simulink model "chapter_3_homework_emulation"  (R2022a)
settings: Solver=VariableStepAuto  StartTime=0.0  StopTime=60  RelTol=1e-3
settings Model: Creator=slack  LastModifiedBy=slack

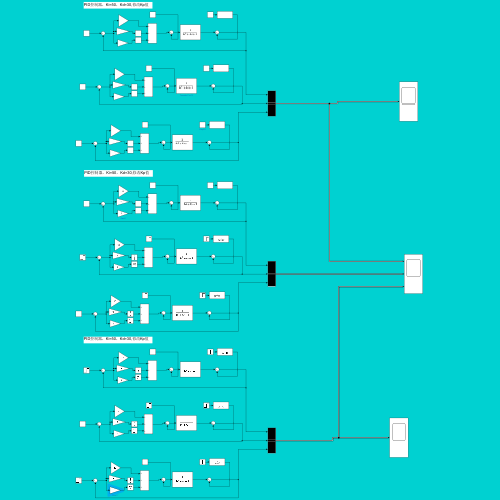
[thumbnail: Simulink's stored preview of the top-level diagram]
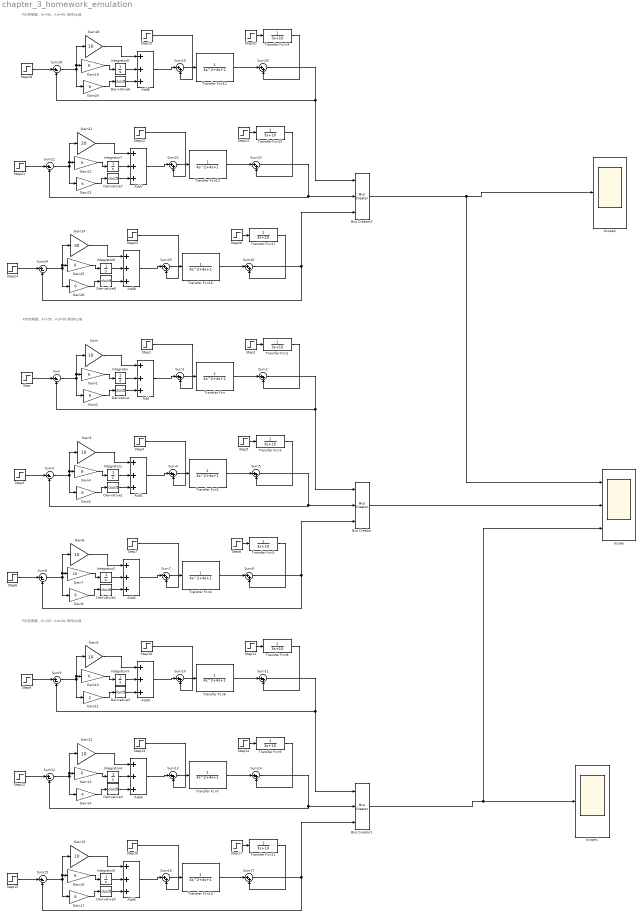
== system chapter_3_homework_emulation ==
  note: PID控制器，Ki=50，Kd=30,修改Kp值
  note: PID控制器，Ki=50，Kd=30,修改Kp值
  note: PID控制器，Ki=50，Kd=30,修改Kp值
  Add{,1..8} (9 alike) : Sum  Inputs=+++
  Bus Creator : BusCreator  Inputs=3
  Bus Creator1 : BusCreator  Inputs=3
  Bus Creator2 : BusCreator  Inputs=3
  Derivative{,1..8} (9 alike) : Derivative
  Gain{,3,6..7,9,12,15,18} (8 alike) : Gain  Gain=10
  Gain{1..2,5,8,10,13,16..17,19..20,22..23,25..26} (14 alike) : Gain  Gain=6
  Gain11 : Gain  Gain=2
  Gain14 : Gain  Gain=4
  Gain21 : Gain  Gain=20
  Gain24 : Gain  Gain=30
  Gain4 : Gain  Gain=8
  Integrator{,1..8} (9 alike) : Integrator
  Scope : Scope  NumInputPorts=3
  Scope1 : Scope
  Scope2 : Scope
  Step{,3,6,9,12,15,18,21,24} (9 alike) : Step  Time=0  After=3  SampleTime=0
  Step{1,4,7,10,13,16,19,22,25} (9 alike) : Step  Time=20  After=6  SampleTime=0
  Step{2,5,8,11,14,17,20,23,26} (9 alike) : Step  Time=40  After=10  SampleTime=0
  Sum{,3,6,9,12,15,18,21,24} (9 alike) : Sum  Inputs=|+-
  Sum{1..2,4..5,7..8,10..11,13..14,16..17,19..20,22..23,25..26} (18 alike) : Sum  Inputs=|++
  Transfer Fcn{,1,4,6..7,10,12..13,16} (9 alike) : TransferFcn  Denominator=[4 4 1]
  Transfer Fcn{2..3,5,8..9,11,14..15,17} (9 alike) : TransferFcn  Denominator=[3 10]
  wires:
  Gain/1 -> Add/1
  Integrator/1 -> Add/2
  Derivative/1 -> Add/3
  Gain1/1 -> Integrator/1
  Gain2/1 -> Derivative/1
  Step/1 -> Sum/1
  Sum/1 -> Gain/1, Gain1/1, Gain2/1
  Sum2/1 -> Bus Creator/1, Sum/2
  Add/1 -> Sum1/1
  Sum1/1 -> Transfer Fcn/1
  Transfer Fcn/1 -> Sum2/1
  Step2/1 -> Transfer Fcn2/1
  Transfer Fcn2/1 -> Sum2/2
  Step1/1 -> Sum1/2
  Derivative1/1 -> Add1/3
  Step5/1 -> Transfer Fcn3/1
  Gain5/1 -> Derivative1/1
  Sum4/1 -> Transfer Fcn1/1
  Gain4/1 -> Integrator1/1
  Step3/1 -> Sum3/1
  Gain3/1 -> Add1/1
  Integrator1/1 -> Add1/2
  Transfer Fcn3/1 -> Sum5/2
  Sum3/1 -> Gain3/1, Gain4/1, Gain5/1
  Add1/1 -> Sum4/1
  Transfer Fcn1/1 -> Sum5/1
  Step4/1 -> Sum4/2
  Sum5/1 -> Sum3/2, Bus Creator/2
  Derivative2/1 -> Add2/3
  Step8/1 -> Transfer Fcn5/1
  Gain8/1 -> Derivative2/1
  Sum7/1 -> Transfer Fcn4/1
  Gain7/1 -> Integrator2/1
  Step6/1 -> Sum6/1
  Gain6/1 -> Add2/1
  Integrator2/1 -> Add2/2
  Transfer Fcn5/1 -> Sum8/2
  Sum6/1 -> Gain6/1, Gain7/1, Gain8/1
  Add2/1 -> Sum7/1
  Transfer Fcn4/1 -> Sum8/1
  Step7/1 -> Sum7/2
  Sum8/1 -> Sum6/2, Bus Creator/3
  Step11/1 -> Transfer Fcn8/1
  Step10/1 -> Sum10/2
  Sum10/1 -> Transfer Fcn6/1
  Gain9/1 -> Add3/1
  Transfer Fcn8/1 -> Sum11/2
  Sum11/1 -> Bus Creator1/1, Sum9/2
  Bus Creator1/1 -> Scope/3, Scope1/1
  Add3/1 -> Sum10/1
  Transfer Fcn7/1 -> Sum14/1
  Gain10/1 -> Integrator3/1
  Add4/1 -> Sum13/1
  Sum12/1 -> Gain12/1, Gain13/1, Gain14/1
  Transfer Fcn9/1 -> Sum14/2
  Integrator4/1 -> Add4/2
  Gain13/1 -> Integrator4/1
  Step14/1 -> Transfer Fcn9/1
  Sum13/1 -> Transfer Fcn7/1
  Derivative3/1 -> Add3/3
  Step12/1 -> Sum12/1
  Gain11/1 -> Derivative3/1
  Integrator3/1 -> Add3/2
  Gain12/1 -> Add4/1
  Step9/1 -> Sum9/1
  Transfer Fcn11/1 -> Sum17/2
  Integrator5/1 -> Add5/2
  Gain15/1 -> Add5/1
  Gain16/1 -> Integrator5/1
  Step15/1 -> Sum15/1
  Sum16/1 -> Transfer Fcn10/1
  Gain14/1 -> Derivative4/1
  Sum9/1 -> Gain9/1, Gain10/1, Gain11/1
  Step17/1 -> Transfer Fcn11/1
  Transfer Fcn6/1 -> Sum11/1
  Gain17/1 -> Derivative5/1
  Derivative5/1 -> Add5/3
  Derivative4/1 -> Add4/3
  Step16/1 -> Sum16/2
  Add5/1 -> Sum16/1
  Sum15/1 -> Gain15/1, Gain16/1, Gain17/1
  Sum17/1 -> Sum15/2, Bus Creator1/3
  Sum14/1 -> Sum12/2, Bus Creator1/2
  Transfer Fcn10/1 -> Sum17/1
  Step13/1 -> Sum13/2
  Step20/1 -> Transfer Fcn14/1
  Step19/1 -> Sum19/2
  Sum19/1 -> Transfer Fcn12/1
  Gain18/1 -> Add6/1
  Transfer Fcn14/1 -> Sum20/2
  Sum20/1 -> Bus Creator2/1, Sum18/2
  Bus Creator2/1 -> Scope/1, Scope2/1
  Add6/1 -> Sum19/1
  Transfer Fcn13/1 -> Sum23/1
  Gain19/1 -> Integrator6/1
  Add7/1 -> Sum22/1
  Sum21/1 -> Gain21/1, Gain22/1, Gain23/1
  Transfer Fcn15/1 -> Sum23/2
  Integrator7/1 -> Add7/2
  Gain22/1 -> Integrator7/1
  Step23/1 -> Transfer Fcn15/1
  Sum22/1 -> Transfer Fcn13/1
  Derivative6/1 -> Add6/3
  Step21/1 -> Sum21/1
  Gain20/1 -> Derivative6/1
  Integrator6/1 -> Add6/2
  Gain21/1 -> Add7/1
  Step18/1 -> Sum18/1
  Transfer Fcn17/1 -> Sum26/2
  Integrator8/1 -> Add8/2
  Gain24/1 -> Add8/1
  Gain25/1 -> Integrator8/1
  Step24/1 -> Sum24/1
  Sum25/1 -> Transfer Fcn16/1
  Gain23/1 -> Derivative7/1
  Sum18/1 -> Gain18/1, Gain19/1, Gain20/1
  Step26/1 -> Transfer Fcn17/1
  Transfer Fcn12/1 -> Sum20/1
  Gain26/1 -> Derivative8/1
  Derivative8/1 -> Add8/3
  Derivative7/1 -> Add7/3
  Step25/1 -> Sum25/2
  Add8/1 -> Sum25/1
  Sum24/1 -> Gain24/1, Gain25/1, Gain26/1
  Sum26/1 -> Sum24/2, Bus Creator2/3
  Sum23/1 -> Sum21/2, Bus Creator2/2
  Transfer Fcn16/1 -> Sum26/1
  Step22/1 -> Sum22/2
  Bus Creator/1 -> Scope/2
